simulink model "ClarkPark"  (R2025b)
settings: Solver=VariableStepAuto  StartTime=0.0  StopTime=10.0  RelTol=1e-3
settings Model: Creator=jff_1  LastModifiedBy=jff_1

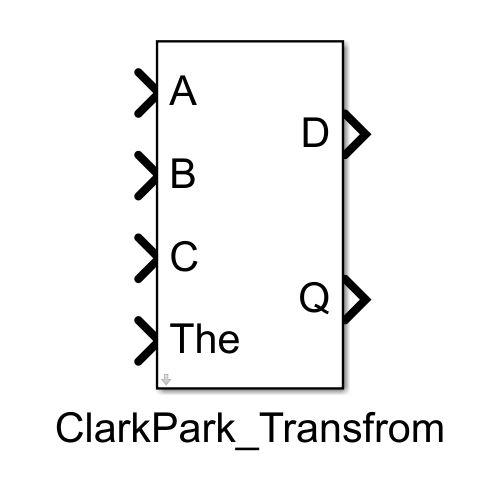
[thumbnail: Simulink's stored preview of the top-level diagram]
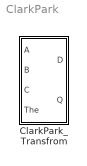
== system ClarkPark ==
  ClarkPark_Transfrom : Subsystem
      mask help:
      | 将三相静止坐标系的 A、B、C 量通过同步旋转角 The(θ) 变换到同步旋转坐标系 d、q。
      | 本模块采用 2/3 幅值不变（amplitude-invariant）系数，常用于电机矢量控制中的电流/电压坐标变换。
      mask Help:
      | 【功能】
      | 把三相静止量 (A,B,C) 变换为同步旋转坐标系的 (d,q)，角度由 The(θ) 提供。
      | 
      | 【输入端口】
      | 
      | A：A 相量（电流/电压等）
      | 
      | B：B 相量
      | 
      | C：C 相量
      | 
      | The：同步旋转角 θ（单位：rad，弧度）
      | 
      | 【输出端口】
      | 
      | D：d 轴分量
      | 
      | Q：q 轴分量
      | 
      | 【计算关系（与模块内部 Fcn 一致）】
      | D = ( Acos(The) + Bcos(The - 2/3pi) + Ccos(The + 2/3pi) ) * 2/3
      | Q = -( Asin(The) + Bsin(The - 2/3pi) + Csin(The + 2/3pi) ) * 2/3
      | 
      | 【说明与注意】
      | 
      | The 必须使用弧度制；若你手里是角度制(°)，请先转换：The = The_deg*pi/180。
      | 
      | 该实现等价于“Clarke(abc→αβ) + Park(αβ→dq)”的组合写法，只是把两步合成到一起。
      | 
      | 若输入三相为对称系统（A+B+C=0），该变换结果最稳定；若含零序分量，本模块未单独输出零序。
      | 
      | 【快速自检建议】
      | 
      | 令 The = 0：此时 D 与 A 的相关性最大，Q 主要由 B/C 组合决定。
      | 
      | 令三相为对称正弦并随 The 同步旋转：理想情况下 d 为常值、q 约为 0（或相反，取决于相位定义）。
      mask DialogControl ParameterGroupVar Prompt: 参数
      mask Display:
      | % 输入端口
      | port_label('input',1,'A');
      | port_label('input',2,'B');
      | port_label('input',3,'C');
      | port_label('input',4,'The');
      | 
      | % 输出端口
      | port_label('output',1,'D');
      | port_label('output',2,'Q');

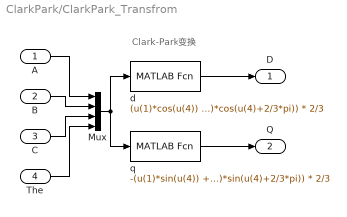
== system ClarkPark/ClarkPark_Transfrom ==
  note: Clark-Park变换
  A : Inport
  B : Inport  Port=2
  C : Inport  Port=3
  The : Inport  Port=4
  Mux : Mux
  d : MATLABFcn  MATLABFcn=(u(1)*cos(u(4)) + u(2)*cos(u(4)-2/3*pi) + u(3)*cos(u(4)+2/3*pi)) * 2/3
  q : MATLABFcn  MATLABFcn=-(u(1)*sin(u(4)) + u(2)*sin(u(4)-2/3*pi) + u(3)*sin(u(4)+2/3*pi)) * 2/3
  D : Outport
  Q : Outport  Port=2
  wires:
  The/1 -> Mux/4
  C/1 -> Mux/3
  B/1 -> Mux/2
  Mux/1 -> q/1, d/1
  q/1 -> Q/1
  d/1 -> D/1
  A/1 -> Mux/1
